simulink model "vmc_velocity_control_loop"  (R2022b)
settings: Solver=VariableStepAuto  StartTime=0.0  StopTime=0.1  RelTol=1e-3
settings Model: Creator=Mahadevu Sudheer  LastModifiedBy=Mahadevu Sudheer

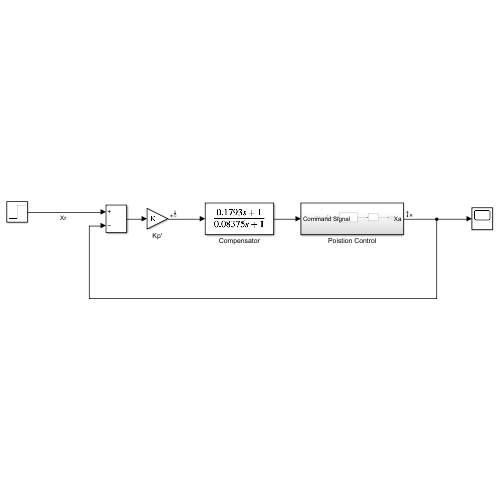
[thumbnail: Simulink's stored preview of the top-level diagram]
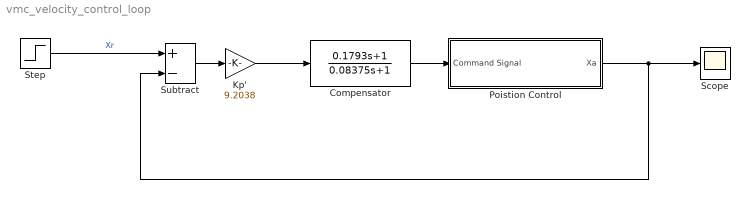
== system vmc_velocity_control_loop ==
  Compensator : TransferFcn  Numerator=[0.1793 1]  Denominator=[0.08375 1]
  Kp' : Gain  Gain=9.2038
  Poistion Control : Subsystem
  Scope : Scope
  Step : Step  Time=0  SampleTime=0
  Subtract : Sum  Inputs=+-
  wires:
  Kp'/1 -> Compensator/1
  Step/1 -> Subtract/1  "Xr"
  Subtract/1 -> Kp'/1
  Poistion Control/1(Xa) -> Subtract/2, Scope/1
  Compensator/1 -> Poistion Control/1(Command Signal)

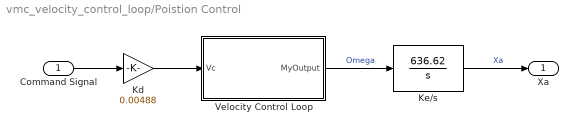
== system vmc_velocity_control_loop/Poistion Control ==
  Command Signal : Inport
  Kd : Gain  Gain=0.00488
  Ke/s : TransferFcn  Numerator=[636.62]  Denominator=[1 0]
  Velocity Control Loop : Subsystem
  Xa : Outport
  wires:
  Ke/s/1 -> Xa/1  "Xa"
  Velocity Control Loop/1(MyOutput) -> Ke/s/1  "Omega"
  Kd/1 -> Velocity Control Loop/1(Vc)
  Command Signal/1 -> Kd/1

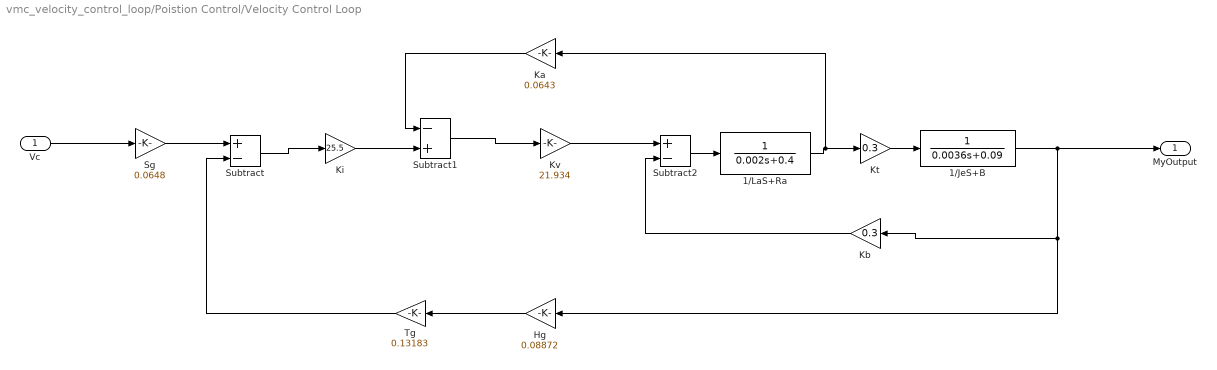
== system vmc_velocity_control_loop/Poistion Control/Velocity Control Loop ==
  Vc : Inport
  1/JeS+B : TransferFcn  Denominator=[0.0036 0.09]
  1/LaS+Ra : TransferFcn  Denominator=[0.002 0.4]
  Hg : Gain  Gain=0.08872
  Ka : Gain  Gain=0.0643
  Kb : Gain  Gain=0.3
  Ki : Gain  Gain=25.5
  Kt : Gain  Gain=0.3
  Kv : Gain  Gain=21.934
  Sg : Gain  Gain=0.0648
  Subtract : Sum  Inputs=+-
  Subtract1 : Sum  Inputs=-+
  Subtract2 : Sum  Inputs=+-
  Tg : Gain  Gain=0.13183
  MyOutput : Outport
  wires:
  1/JeS+B/1 -> MyOutput/1, Kb/1, Hg/1
  Tg/1 -> Subtract/2
  Subtract2/1 -> 1/LaS+Ra/1
  Kb/1 -> Subtract2/2
  1/LaS+Ra/1 -> Ka/1, Kt/1
  Sg/1 -> Subtract/1
  Kt/1 -> 1/JeS+B/1
  Kv/1 -> Subtract2/1
  Subtract1/1 -> Kv/1
  Subtract/1 -> Ki/1
  Ka/1 -> Subtract1/1
  Ki/1 -> Subtract1/2
  Hg/1 -> Tg/1
  Vc/1 -> Sg/1
